simulink model "TankLevelEstimator_SimplifiedNonlinear_Simulink"  (R2020b)
settings: Solver=VariableStepAuto  StartTime=0.0  StopTime=25  RelTol=1e-3
values from neighbouring files (symbols this model uses):
  t_step = 1    [TankLevelEstimator_SimplifiedLinear.m]
libraries: simulink x2, cstblocks x1
settings Model: Creator=Jonas  LastModifiedBy=Jonas

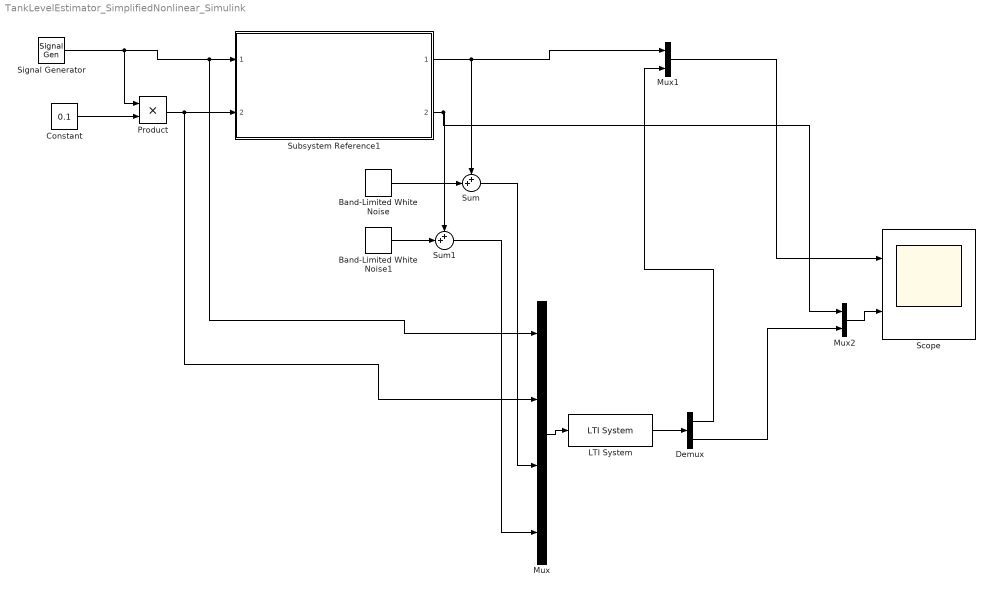
== system TankLevelEstimator_SimplifiedNonlinear_Simulink ==
  Band-Limited White Noise : simulink/Sources/Band-Limited White Noise  Cov=0.1  Ts=t_step  seed=[23341]
  Band-Limited White Noise1 : simulink/Sources/Band-Limited White Noise  Cov=0.1  Ts=t_step  seed=[23341]
  Constant : Constant  Value=0.1
  Demux : Demux  Outputs=2
  LTI System : cstblocks/LTI System  sys=sys_obsv  IC=[]
  Mux : Mux
  Mux1 : Mux  Inputs=2
  Mux2 : Mux  Inputs=2
  Product : Product
  Scope : Scope  NumInputPorts=2
  Signal Generator : SignalGenerator  Frequency=1/(10*t_step)
  Subsystem Reference1 : Subsystem  ReferencedSubsystem=TankLevelDynamics_SimplifiedNonlinear_Simulink
  Sum : Sum  Inputs=++|
  Sum1 : Sum  Inputs=++|
  wires:
  Mux2/1 -> Scope/2
  Demux/1 -> Mux1/2
  Demux/2 -> Mux2/2
  Subsystem Reference1/2 -> Sum1/1, Mux2/1
  Mux/1 -> LTI System/1
  Sum1/1 -> Mux/4
  Signal Generator/1 -> Product/1, Subsystem Reference1/1, Mux/1
  LTI System/1 -> Demux/1
  Band-Limited White Noise/1 -> Sum/2
  Band-Limited White Noise1/1 -> Sum1/2
  Mux1/1 -> Scope/1
  Product/1 -> Subsystem Reference1/2, Mux/2
  Sum/1 -> Mux/3
  Constant/1 -> Product/2
  Subsystem Reference1/1 -> Mux1/1, Sum/1
